simulink model "HeartCFGs"  (R2024b)
settings: Solver=VariableStepAuto  StartTime=0.0  StopTime=10.0  RelTol=1e-3
settings Model: Creator=ball907  LastModifiedBy=ball907

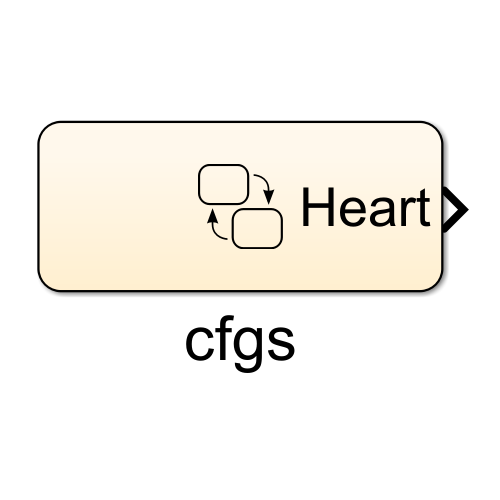
[thumbnail: Simulink's stored preview of the top-level diagram]
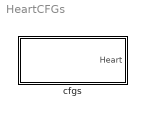
== system HeartCFGs ==
  cfgs : Stateflow chart  TreatAsAtomicUnit=on

== stateflow chart HeartCFGs/cfgs ==
  settings: executeAtInitialization=1
  state Ini
  (default) -> Ini : {Heart=cfgdata;}
  data: Heart output; cfgdata_second parameter
